simulink model "stable"  (R2016b)
settings: Solver=VariableStepAuto  StartTime=0.0  StopTime=20.0  RelTol=1e-3
settings Model: Creator=gz199  LastModifiedBy=gz199

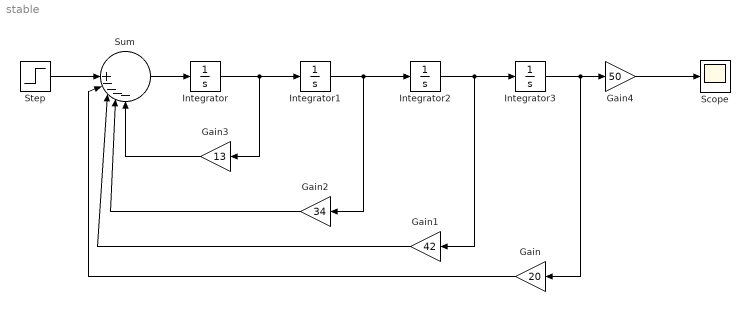
== system stable ==
  Gain : Gain  Gain=20
  Gain1 : Gain  Gain=42
  Gain2 : Gain  Gain=34
  Gain3 : Gain  Gain=13
  Gain4 : Gain  Gain=50
  Integrator{,1..3} (4 alike) : Integrator
  Scope : Scope
  Step : Step  Time=0  SampleTime=0
  Sum : Sum  Inputs=||||+----
  wires:
  Integrator/1 -> Gain3/1, Integrator1/1
  Integrator1/1 -> Gain2/1, Integrator2/1
  Integrator2/1 -> Gain1/1, Integrator3/1
  Sum/1 -> Integrator/1
  Gain/1 -> Sum/2
  Gain3/1 -> Sum/5
  Gain2/1 -> Sum/4
  Gain1/1 -> Sum/3
  Integrator3/1 -> Gain4/1, Gain/1
  Step/1 -> Sum/1
  Gain4/1 -> Scope/1
